simulink model "untitled1"  (R2024b)
settings: Solver=ode15s  StartTime=0.0  StopTime=5  RelTol=1e-3
undefined symbols (not defined in the file): Ion, Lithium
libraries: spsDiodeLib x9, spsSeriesRLCBranchLib x6, spsMosfetLib x5, spsACVoltageSourceLib x1, spsBatteryLib x1, spsLinearTransformerLib x1, spsVoltageMeasurementLib x1, sps_lib x1
settings Model: Creator=Niksh  LastModifiedBy=Niksh

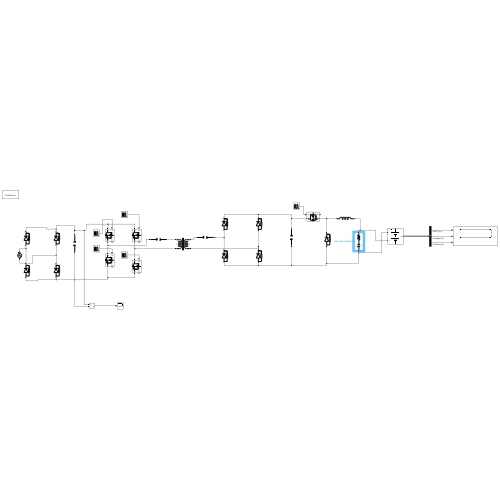
[thumbnail: Simulink's stored preview of the top-level diagram]
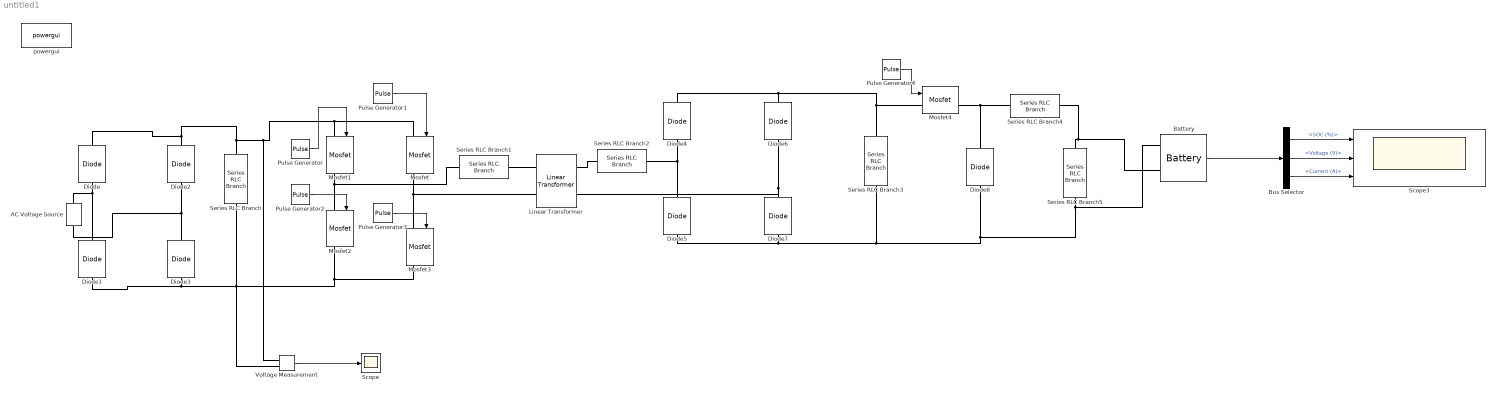
== system untitled1 ==
  AC Voltage Source : spsACVoltageSourceLib/AC Voltage Source  Amplitude=230  Phase=0  Frequency=60  SampleTime=0  Measurements=None  BusType=swing  Pref=10e3  Qref=0  Qmin=-inf  Qmax=+inf
  Battery : spsBatteryLib/Battery  BatType=Lithium-Ion  NomV=50  NomQ=6.5  SOC=75  Batt_Tr=30  PresetModel=on  MaxQ=6.5  MinV=37.5  FullV=58.1994  Dis_rate=2.8261  R=0.076923  Normal_OP=5.8783  expZone="[54.0193     0.319348]"
  Bus Selector : BusSelector  OutputSignals=SOC (%),Voltage (V),Current (A)
  Diode{,1..8} (9 alike) : spsDiodeLib/Diode  Ron=0.001  Lon=0  Vf=0.8  IC=0  UseSnubber=0  Rs=500  Cs=250e-9  Measurements=off
  Linear Transformer : spsLinearTransformerLib/Linear Transformer  UNITS=pu  NominalPower=[ 250e6 50]  winding1=[230 0.002 0.08]  winding2="[160  0.002  0.08 ]"  ThreeWindings=off  winding3=[ 315e3 0.002 0.08 ]  RmLm=[ 500 500 ]  Measurements=None  DataType=off
  Mosfet{,1..4} (5 alike) : spsMosfetLib/Mosfet  Ron=0.1  Lon=0  Rd=0.01  Vfd=0  IC=0  Rs=1e5  Cs=inf  Measurements=on
  Pulse Generator : DiscretePulseGenerator  PulseType=Time based  Period=0.02  PulseWidth=50
  Pulse Generator1 : DiscretePulseGenerator  PulseType=Time based  Period=0.02  PulseWidth=50  PhaseDelay=0.01
  Pulse Generator2 : DiscretePulseGenerator  PulseType=Time based  Period=0.02  PulseWidth=50  PhaseDelay=0.01
  Pulse Generator3 : DiscretePulseGenerator  PulseType=Time based  Period=0.02  PulseWidth=50
  Pulse Generator4 : DiscretePulseGenerator  PulseType=Time based  Period=0.02  PulseWidth=50
  Scope : Scope
  Scope3 : Scope  NumInputPorts=3
  Series RLC Branch : spsSeriesRLCBranchLib/Series RLC Branch  LConnTagsString=__new0  RConnTagsString=__new0  BranchType=C  Resistance=1  Inductance=1e-3  SetiL0=off  InitialCurrent=0  Capacitance=1000e-6  Setx0=off  InitialVoltage=0  Measurements=None
  Series RLC Branch1 : spsSeriesRLCBranchLib/Series RLC Branch  LConnTagsString=__new0  RConnTagsString=__new0  BranchType=C  Resistance=1  Inductance=1e-3  SetiL0=off  InitialCurrent=0  Capacitance=4.9e-3  Setx0=off  InitialVoltage=0  Measurements=None
  Series RLC Branch2 : spsSeriesRLCBranchLib/Series RLC Branch  LConnTagsString=__new0  RConnTagsString=__new0  BranchType=C  Resistance=1  Inductance=1e-3  SetiL0=off  InitialCurrent=0  Capacitance=4.9e-3  Setx0=off  InitialVoltage=0  Measurements=None
  Series RLC Branch3 : spsSeriesRLCBranchLib/Series RLC Branch  LConnTagsString=__new0  RConnTagsString=__new0  BranchType=C  Resistance=1  Inductance=1e-3  SetiL0=off  InitialCurrent=0  Capacitance=1000e-6  Setx0=off  InitialVoltage=0  Measurements=None
  Series RLC Branch4 : spsSeriesRLCBranchLib/Series RLC Branch  LConnTagsString=__new0  RConnTagsString=__new0  BranchType=L  Resistance=1  Inductance=75e-3  SetiL0=off  InitialCurrent=0  Capacitance=1000e-6  Setx0=off  InitialVoltage=0  Measurements=None
  Series RLC Branch5 : spsSeriesRLCBranchLib/Series RLC Branch  LConnTagsString=__new0  RConnTagsString=__new0  BranchType=RC  Resistance=0.001  Inductance=1e-3  SetiL0=off  InitialCurrent=0  Capacitance=100e-3  Setx0=off  InitialVoltage=0  Measurements=None
  Voltage Measurement : spsVoltageMeasurementLib/Voltage Measurement  PhasorSimulation=off  OutputType=Complex  PSBequivalent=0
  powergui : sps_lib/powergui  Priority=1  SimulationMode=Continuous  SampleTime=50e-6  frequency=60  Iterations=50  frequencyindice=0  Pbase=100e6  ErrMax=1e-4  UnitsV=kV  UnitsW=MW  buscounter=0  FunctionMessages=off  echomessages=off  EnableUseOfTLC=off  CurrentSourceSwitches=off  DisableSnubberDevices=off  DisableRonSwitches=off  DisableVfSwitches=off  DisplayEquations=off  AutomaticDiscreteSolvers=off  SolverType=Tustin/Backward Euler (TBE)  Interpol=off  ExternalGateDelay=off  methode=off  Ts=100  x0status=blocks  SPID=on  SwTol=0  HookPort=off  NonlinearTolerance=1e-4  nMaxIteration=100  ContinueOnMaxIteration=off  RestoreLinks=warning  ResistiveCurrentMeasurement=off  Frange=[0:2:500]  Ylog=off  Xlog=on  ShowGrid=off  save=off  variable=ZData  structure=0  ZoomFFT=off  StartTime=0.0  cycles=1  DisplayStyle=1  fundamental=60  FreqAxis=off  MaxFrequency=1000  frequencyindicesteady=1  RmsSteady=1  display=off
  wires:
  Voltage Measurement/1 -> Scope/1
  Pulse Generator/1 -> Mosfet1/1
  Pulse Generator3/1 -> Mosfet3/1
  Pulse Generator2/1 -> Mosfet2/1
  Pulse Generator4/1 -> Mosfet4/1
  Battery/1 -> Bus Selector/1
  Bus Selector/1 -> Scope3/1  "<SOC (%)>"
  Bus Selector/3 -> Scope3/3  "<Current (A)>"
  Bus Selector/2 -> Scope3/2  "<Voltage (V)>"
  Pulse Generator1/1 -> Mosfet/1
  connections:
  Diode/RConn1 -- Mosfet/LConn1 -- Mosfet1/LConn1 -- Voltage Measurement/LConn1 -- Series RLC Branch/LConn1 -- Diode2/RConn1
  Diode2/LConn1 -- AC Voltage Source/LConn1 -- Diode3/RConn1
  Diode1/RConn1 -- AC Voltage Source/RConn1 -- Diode/LConn1
  Diode1/LConn1 -- Mosfet3/RConn1 -- Mosfet2/RConn1 -- Series RLC Branch/RConn1 -- Voltage Measurement/LConn2 -- Diode3/LConn1
  Mosfet2/LConn1 -- Series RLC Branch1/RConn1 -- Mosfet1/RConn1
  Mosfet3/LConn1 -- Linear Transformer/LConn2 -- Mosfet/RConn1
  Series RLC Branch1/LConn1 -- Linear Transformer/LConn1
  Series RLC Branch2/RConn1 -- Linear Transformer/RConn1
  Diode6/LConn1 -- Linear Transformer/RConn2 -- Diode7/RConn1
  Diode4/RConn1 -- Series RLC Branch3/LConn1 -- Mosfet4/LConn1 -- Diode6/RConn1
  Diode5/RConn1 -- Series RLC Branch2/LConn1 -- Diode4/LConn1
  Diode7/LConn1 -- Diode8/LConn1 -- Battery/LConn2 -- Series RLC Branch5/RConn1 -- Series RLC Branch3/RConn1 -- Diode5/LConn1
  Mosfet4/RConn1 -- Series RLC Branch4/LConn1 -- Diode8/RConn1
  Series RLC Branch4/RConn1 -- Battery/LConn1 -- Series RLC Branch5/LConn1
